simulink model "tx"  (R2019a)
settings: Solver=VariableStepAuto  StartTime=0.0  StopTime=10  RelTol=1e-3
undefined symbols (not defined in the file): fdesignblkfcn, gcbh
libraries: commnoisgen2 x1, dspobslib x1
(part 2 of 2)

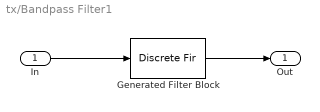
== system tx/Bandpass Filter1 ==
  In : Inport
  Generated Filter Block : DiscreteFir  Tag=BlockMethodSubSystem  Coefficients=[0.000877708768380303984 -1.05600530367274152e-05 -1.06096719831617892e-05 -1.08346193913756847e-05 -1.10786126885892939e-05 -1.14932293063446439e-05 -1.19199472524715491e-05 -1.25116094910030125e-05 -1.31058587664196471e-05 -1.38584613502859381e-05 -1.46012717847146794e-05 -1.5496357900643843e-05 -1.63648080606204182e-05 -1.73839298442266194e-05 -1.83494041037087982e-05 -1.94945886191615503e-05 -2.18649645451131792e-05 -2.1064413781133706e-05 -2.23586533866838334e-05 -2.36208161710170766e-05 -2.48592448294064367e-05 -2.61109840215829458e-05 -2.73152004359089508e-05 -2.85328124920062416e-05 -2.96876017605783539e-05 -3.08477108718814043e-05 -3.19327419838016891e-05 -3.30111062742944857e-05 -3.40051042403866511e-05 -3.49763742021249463e-05 -3.58599931045616499e-05 -3.66898517969579605e-05 -3.71592730296003808e-05 -3.84238580850499497e-05 -3.88703901532032412e-05 -3.93607032269104084e-05 -3.97123477061159767e-05 -4.00552088324267154e-05 -4.02539554211982882e-05 -4.04250253497524283e-05 -4.04469370915386695e-05 -4.0431213970025027e-05 -4.02637367705020472e-05 -4.00544864010071245e-05 -3.9692658316945904e-05 -3.92907343010702372e-05 -3.87348551995032398e-05 -3.81526648822992382e-05 -3.75106260358264079e-05 -3.64811073327381752e-05 -3.56878671192981979e-05 -3.47818599766077253e-05 -3.37577078993430216e-05 -3.26731274112494014e-05 -3.14897712788517626e-05 -3.0269063522924528e-05 -2.89676661855913604e-05 -2.76455800095741933e-05 -2.62601077049361793e-05 -2.48679478975368613e-05 -2.34303846104704904e-05 -2.19979937798261711e-05 -2.05409287241194085e-05 -1.90946528930930953e-05 -1.76060431218239086e-05 -1.63303077578821681e-05 -1.48286603092871077e-05 -1.3451502596984583e-05 -1.20954792401510884e-05 -1.08304079263699593e-05 -9.59175466211999606e-06 -8.44387680901548948e-06 -7.33350625715587217e-06 -6.32143311714381678e-06 -5.35947016632842398e-06 -4.5052157282076755e-06 -3.71212714646285396e-06 -3.03636080601569613e-06 -2.42868559687013999e-06 -1.95031207691315992e-06 -1.56122292285819971e-06 -1.19783453975661792e-06 -1.07363565950082014e-06 -1.00421652751909226e-06 -1.01958633202297103e-06 -1.13607502137897179e-06 -1.34684181686106196e-06 -1.66325789571731501e-06 -2.07046782915276239e-06 -2.5756213411561469e-06 -3.16212639751899203e-06 -3.83342611538371649e-06 -4.57400125994161452e-06 -5.38238525686152505e-06 -6.24742980762690425e-06 -7.15764331491884533e-06 -8.10227638879852403e-06 -9.13574307982853093e-06 -1.00764671777239453e-05 -1.1091197558923396e-05 -1.20993697734882036e-05 -1.31081570307100062e-05 -1.40778099794978961e-05 -1.50167052604025615e-05 -1.58939966163800309e-05 -1.6716686927849625e-05 -1.7456274829059904e-05 -1.81181726780026663e-05 -1.86740938369896019e-05 -1.91297209786242409e-05 -1.9454686389764708e-05 -1.96599605161716954e-05 -1.9713391041999216e-05 -1.958637256532596e-05 -1.93681732782864354e-05 -1.89258471089706832e-05 -1.83016746514769093e-05 -1.74862801218898106e-05 -1.64816452902360067e-05 -1.52763018096280104e-05 -1.38676518244816322e-05 -1.22470320198600231e-05 -1.04138189119970482e-05 -8.36278828312013358e-06 -6.09681629623192063e-06 -3.61272831534917033e-06 -9.18700216958885478e-07 1.99034874265270265e-06 5.09954252008208101e-06 8.38825600489882719e-06 1.19239355304704212e-05 1.55901514914201077e-05 1.94361125866021047e-05 2.34372663654394296e-05 2.75966781079746773e-05 3.18835491122479876e-05 3.62939556853447308e-05 4.07961013905999703e-05 4.53848236121827788e-05 5.00268663763286416e-05 5.47164903182575761e-05 5.94171207481261014e-05 6.41238659790699427e-05 6.87934054179223679e-05 7.34244427192762717e-05 7.79837858963194864e-05 8.24090728391657732e-05 8.67450491967880792e-05 9.09240961548982108e-05 9.49171914765112139e-05 9.87014932157603093e-05 0.000102248351696631982 0.000105538641736135116 0.000108539924500029102 0.000111233369299261605 0.000113585004319728417 0.000115577380720460429 0.000117177714033271521 0.000118369630455673891 0.00011912528763238187 0.000119427214654318158 0.000119243121016593227 ...(+38148 chars)]  InputProcessing=Columns as channels (frame based)
  Out : Outport
  wires:
  In/1 -> Generated Filter Block/1
  Generated Filter Block/1 -> Out/1
